simulink model "RBFNN_Position_PID_Attitude"  (R2018a)
settings: Solver=FixedStepAuto  StartTime=0.0  StopTime=60  FixedStep=1e-3  RelTol=1e-3
settings Model: Creator=hellb  LastModifiedBy=hellb

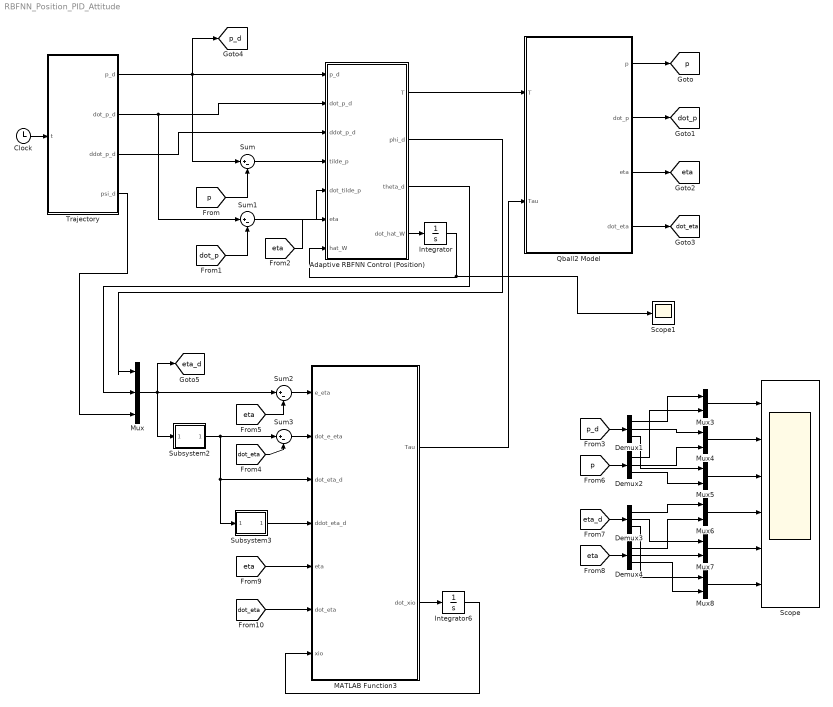
== system RBFNN_Position_PID_Attitude ==
  Adaptive RBFNN Control (Position) : MATLAB Function  TreatAsAtomicUnit=on
  Clock : Clock
  Demux{1..4} (4 alike) : Demux  Outputs=3
  Integrator : Integrator  InitialCondition=0.005*ones(7,3)
  Integrator6 : Integrator  InitialCondition=[0;0;0]
  MATLAB Function3 : MATLAB Function  TreatAsAtomicUnit=on
  Mux : Mux  Inputs=3
  Mux{3..8} (6 alike) : Mux  Inputs=2
  Qball2 Model : Subsystem
  Scope : Scope  NumInputPorts=6
  Scope1 : Scope
  Subsystem2 : Subsystem
  Subsystem3 : Subsystem
  Sum{,1..3} (4 alike) : Sum  Inputs=|+-
  Trajectory : MATLAB Function  TreatAsAtomicUnit=on
  tag scope: dot_eta=global, dot_p=global, eta=global, eta_d=global, p=global, p_d=global
  wires:
  Qball2 Model/3(eta) -> [eta]
  Demux3/3 -> Mux8/1
  Demux2/3 -> Mux5/2
  Integrator/1 -> Scope1/1, Adaptive RBFNN Control (Position)/7(hat_W)
  Demux4/2 -> Mux7/2
  Demux2/2 -> Mux4/2
  Demux1/2 -> Mux4/1
  Demux1/1 -> Mux3/1
  Demux4/1 -> Mux6/2
  Mux4/1 -> Scope/2
  [eta_d] -> Demux3/1
  [p] -> Demux2/1
  Qball2 Model/4(dot_eta) -> [dot_eta]
  Trajectory/3(ddot_p_d) -> Adaptive RBFNN Control (Position)/3(ddot_p_d)
  Demux1/3 -> Mux5/1
  Demux3/2 -> Mux7/1
  Mux3/1 -> Scope/1
  Sum/1 -> Adaptive RBFNN Control (Position)/4(tilde_p)
  Mux5/1 -> Scope/3
  Adaptive RBFNN Control (Position)/4(dot_hat_W) -> Integrator/1
  Sum1/1 -> Adaptive RBFNN Control (Position)/5(dot_tilde_p)
  Clock/1 -> Trajectory/1(t)
  Qball2 Model/1(p) -> [p]
  Mux6/1 -> Scope/4
  Demux2/1 -> Mux3/2
  [p_d] -> Demux1/1
  Demux4/3 -> Mux8/2
  Qball2 Model/2(dot_p) -> [dot_p]
  Mux8/1 -> Scope/6
  [eta] -> Adaptive RBFNN Control (Position)/6(eta)
  Trajectory/2(dot_p_d) -> Sum1/1, Adaptive RBFNN Control (Position)/2(dot_p_d)
  Demux3/1 -> Mux6/1
  [eta] -> Demux4/1
  [p] -> Sum/2
  [dot_p] -> Sum1/2
  Trajectory/1(p_d) -> [p_d], Sum/1, Adaptive RBFNN Control (Position)/1(p_d)
  Mux7/1 -> Scope/5
  Adaptive RBFNN Control (Position)/1(T) -> Qball2 Model/1(T)
  [dot_eta] -> Sum3/2
  Subsystem3/1(Out1) -> MATLAB Function3/4(ddot_eta_d)
  [eta] -> Sum2/2
  [eta] -> MATLAB Function3/5(eta)
  MATLAB Function3/1(Tau) -> Qball2 Model/2(Tau)
  Sum3/1 -> MATLAB Function3/2(dot_e_eta)
  [dot_eta] -> MATLAB Function3/6(dot_eta)
  Mux/1 -> [eta_d], Subsystem2/1(In1), Sum2/1
  Sum2/1 -> MATLAB Function3/1(e_eta)
  Subsystem2/1(Out1) -> Sum3/1, Subsystem3/1(In1), MATLAB Function3/3(dot_eta_d)
  Integrator6/1 -> MATLAB Function3/7(xio)
  MATLAB Function3/2(dot_xio) -> Integrator6/1
  Adaptive RBFNN Control (Position)/3(theta_d) -> Mux/2
  Adaptive RBFNN Control (Position)/2(phi_d) -> Mux/1
  Trajectory/4(psi_d) -> Mux/3

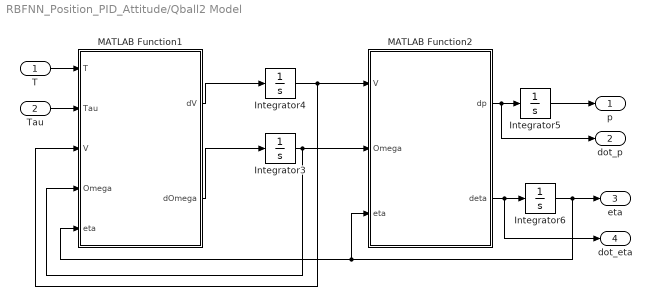
== system RBFNN_Position_PID_Attitude/Qball2 Model ==
  T : Inport
  Tau : Inport  Port=2
  Integrator3 : Integrator  InitialCondition=[0;0;0]
  Integrator4 : Integrator  InitialCondition=[0;0;0]
  Integrator5 : Integrator  InitialCondition=[0;0;0.3]  LimitOutput=on  UpperSaturationLimit=[inf;inf;inf]  LowerSaturationLimit=[-inf;-inf;0.3]
  Integrator6 : Integrator  InitialCondition=[0;0;0]
  MATLAB Function1 : MATLAB Function  TreatAsAtomicUnit=on
  MATLAB Function2 : MATLAB Function  TreatAsAtomicUnit=on
  p : Outport
  dot_p : Outport  Port=2
  eta : Outport  Port=3
  dot_eta : Outport  Port=4
  wires:
  MATLAB Function2/2(deta) -> Integrator6/1, dot_eta/1
  MATLAB Function2/1(dp) -> dot_p/1, Integrator5/1
  MATLAB Function1/1(dV) -> Integrator4/1
  MATLAB Function1/2(dOmega) -> Integrator3/1
  Tau/1 -> MATLAB Function1/2(Tau)
  T/1 -> MATLAB Function1/1(T)
  Integrator6/1 -> eta/1, MATLAB Function2/3(eta), MATLAB Function1/5(eta)
  Integrator5/1 -> p/1
  Integrator3/1 -> MATLAB Function1/4(Omega), MATLAB Function2/2(Omega)
  Integrator4/1 -> MATLAB Function1/3(V), MATLAB Function2/1(V)

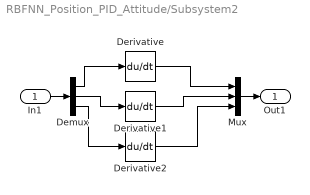
== system RBFNN_Position_PID_Attitude/Subsystem2 ==
  In1 : Inport
  Demux : Demux  Outputs=3
  Derivative : Derivative
  Derivative1 : Derivative
  Derivative2 : Derivative
  Mux : Mux  Inputs=3
  Out1 : Outport
  wires:
  In1/1 -> Demux/1
  Demux/1 -> Derivative/1
  Mux/1 -> Out1/1
  Demux/2 -> Derivative1/1
  Demux/3 -> Derivative2/1
  Derivative1/1 -> Mux/2
  Derivative/1 -> Mux/1
  Derivative2/1 -> Mux/3

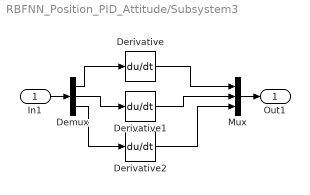
== system RBFNN_Position_PID_Attitude/Subsystem3 ==
  In1 : Inport
  Demux : Demux  Outputs=3
  Derivative : Derivative
  Derivative1 : Derivative
  Derivative2 : Derivative
  Mux : Mux  Inputs=3
  Out1 : Outport
  wires:
  Derivative2/1 -> Mux/3
  Derivative/1 -> Mux/1
  Derivative1/1 -> Mux/2
  Demux/3 -> Derivative2/1
  Demux/2 -> Derivative1/1
  Mux/1 -> Out1/1
  Demux/1 -> Derivative/1
  In1/1 -> Demux/1

== matlab function RBFNN_Position_PID_Attitude/Trajectory ==
  data: t input; p_d output; dot_p_d output; ddot_p_d output; psi_d output
function [p_d,dot_p_d,ddot_p_d,psi_d] = fcn(t)

x_amp = 0.5;
y_amp = 1;
% z_amp = 0;

x_frec = 2*pi/4;
y_frec = 2*pi/8;
% z_frec = 0;

z_b = 1;

p_d = [x_amp*sin(x_frec*t);
       y_amp*cos(y_frec*t);
       z_b];
   
dot_p_d = [x_frec*x_amp*cos(x_frec*t);
           y_frec*y_amp*-sin(y_frec*t);
           0];
       
ddot_p_d = [x_frec^2*x_amp*-sin(x_frec*t);
            y_frec^2*y_amp*-cos(y_frec*t);
            0];
        
psi_d = 0;

== matlab function RBFNN_Position_PID_Attitude/Adaptive RBFNN Control (Position) ==
  data: T output; p_d input; dot_p_d input; ddot_p_d input; tilde_p input; phi_d output; theta_d output; dot_hat_W output; dot_tilde_p input; eta input; hat_W input
function [T, phi_d,theta_d,dot_hat_W] = fcn(p_d, dot_p_d, ddot_p_d, tilde_p, dot_tilde_p, eta, hat_W)
m = 1.79;
g = 9.81;
%% RBFNN parameters
c      = [-1.5,-1,-0.5,0,0.5,1,1.5];
J      = length(c);
sigma  = 5*ones(J,1);
Lambda = 0.85;
A      = 10;
Kv     = 12;
%%
phi   = eta(1);
theta = eta(2);
psi   = eta(3);

M  = diag([1/m 1/m cos(phi)*cos(theta)/m]);
e3 = [0;0;1];

Xin = [tilde_p' dot_tilde_p' p_d' dot_p_d' ddot_p_d'];
P = zeros(J,1);
for i=1:J
    P(i) = exp(-(norm(Xin - c(i))^2)/sigma(i)^2);
end

gamma = dot_tilde_p + Lambda*tilde_p;

dot_hat_W = A*P*gamma';
hat_f = hat_W'*P;
u = M\(g*e3 + hat_f + Kv*gamma);

u1 = u(1)/u(3);
u2 = u(2)/u(3);

T = u(3);

phi_d   = asin(u1*sin(psi) - u2*cos(psi));
theta_d = asin((u1*cos(psi) + u2*sin(psi))/cos(phi_d));

== matlab function RBFNN_Position_PID_Attitude/MATLAB Function3 ==
  data: e_eta input; dot_e_eta input; dot_eta_d input; ddot_eta_d input; eta input; Tau output; dot_eta input; xio input; dot_xio output
function [Tau, dot_xio] = fcn(e_eta, dot_e_eta, dot_eta_d, ddot_eta_d, eta, dot_eta, xio)

% Kpo = 8*diag([1;1;1]);
% Kdo = 0.2*diag([1;1;1]);
% Kio = 0.05*diag([1;1;1]);

Kpo = 2*diag([1;1;1]);
Kdo = 0.5*diag([1;1;1]);
Kio = 0.015*diag([1;1;1]);

alpha = 1;
beta  = 1;

Ixx = 0.03;
Iyy = 0.03;
Izz = 0.04;

phi   = eta(1);
theta = eta(2);

W = [1 sin(phi)*tan(theta) cos(phi)*tan(theta)
     0 cos(phi)          -sin(phi)
     0 sin(phi)/cos(theta) cos(phi)/cos(theta)];

iW = [1 0         -sin(theta)
      0 cos(phi)  cos(theta)*sin(phi)
      0 -sin(phi) cos(theta)*cos(phi)];

dW = [0 cos(phi)*tan(theta)+sin(phi)*sec(theta)^2          -sin(phi)*tan(theta)+cos(phi*sec(theta)^2)
      0 -sin(phi)                                          -cos(phi)
      0 cos(phi)*sec(theta)+sin(phi)*sec(theta)*tan(theta) -sin(phi)*sec(theta)+cos(phi)*tan(theta)+cos(phi)*sec(theta)*tan(theta)];
  
I = diag([Ixx Iyy Izz]);

iWdeta = iW*dot_eta;

SiWdeta = [ 0         -iWdeta(3)  iWdeta(2)
            iWdeta(3)  0         -iWdeta(1)
           -iWdeta(2)  iWdeta(1)  0];

Ho = iW'*I*iW;
Co = iW'*(SiWdeta*I - I*iW*dW)*iW;

fo      = Ho*ddot_eta_d + Co*dot_eta_d + Kpo*e_eta + Kdo*dot_e_eta + Kio*xio;
Tau     = W'*fo;
dot_xio = alpha*e_eta + beta*dot_e_eta;

== matlab function RBFNN_Position_PID_Attitude/Qball2 Model/MATLAB Function1 ==
  data: T input; Tau input; V input; dV output; Omega input; eta input; dOmega output
function [dV,dOmega] = fcn(T,Tau,V,Omega,eta)

%  TTA = [1.7613 %Parametros identificados 1
%     0.0128
%     0.0151
%     0.0024];

%  TTA = [1.7874 %Parametros identificados 2
%     0.0156
%     0.0186
%     0.0010];

%  TTA = [1.7917 %Parametros identificados 3
%     0.0140
%     0.0148
%     0.0013];

 TTA = [1.79 %Parametros fabricante
    0.03
    0.03
    0.04];

TAUphi = Tau(1);
TAUtta = Tau(2);
TAUpsi = Tau(3);

u = V(1);
v = V(2);
w = V(3);

p = Omega(1);
q = Omega(2);
r = Omega(3);

phi = eta(1);
tta = eta(2);

gbx = -9.8*sin(tta);
gby = 9.8*cos(tta)*sin(phi);
gbz = 9.8*cos(tta)*cos(phi);

  m = TTA(1,1);
Ixx = TTA(2,1);
Iyy = TTA(3,1);
Izz = TTA(4,1);

du = r*v - q*w - gbx;
dv = p*w - r*u - gby;
dw = q*u - p*v - gbz + T/m;
dp = ((Iyy-Izz)*q*r + TAUphi)/Ixx;
dq = ((Izz-Ixx)*p*r + TAUtta)/Iyy;
dr = ((Ixx-Iyy)*p*q + TAUpsi)/Izz;

    dV = [du;dv;dw];
dOmega = [dp;dq;dr];

== matlab function RBFNN_Position_PID_Attitude/Qball2 Model/MATLAB Function2 ==
  data: V input; dp output; Omega input; eta input; deta output
function [dp,deta] = fcn(V,Omega,eta)

phi = eta(1);
tta = eta(2);
psi = eta(3);

R = [cos(psi)*cos(tta)  -sin(psi)*cos(phi)+cos(psi)*sin(tta)*sin(phi)   sin(psi)*sin(phi)+cos(psi)*cos(phi)*sin(tta)
     sin(psi)*cos(tta)   cos(psi)*cos(phi)+sin(phi)*sin(tta)*sin(psi)   sin(tta)*sin(psi)*cos(phi)-cos(psi)*sin(phi)
     -sin(tta)           cos(tta)*sin(phi)                              cos(tta)*cos(phi)];
 
W = [1  sin(phi)*tan(tta)   cos(phi)*tan(tta)
     0  cos(phi)           -sin(phi)
     0  sin(phi)/cos(tta)   cos(phi)/cos(tta)];

dp = R*V;
deta = W*Omega;
